simulink model "TestFun_2017"  (R2017a)
settings: Solver=VariableStepAuto  StartTime=0.0  StopTime=5  MaxStep=1e-3  RelTol=1e-3
undefined symbols (not defined in the file or in its folder): Evaluate_Trajectory
settings Model: Creator=Roberto Strada  LastModifiedBy=Davide
settings DataIOCC: ReturnWorkspaceOutputs=on
settings SFSimCC: SimUseLocalCustomCode=on
settings RTWCC: RTWUseLocalCustomCode=on

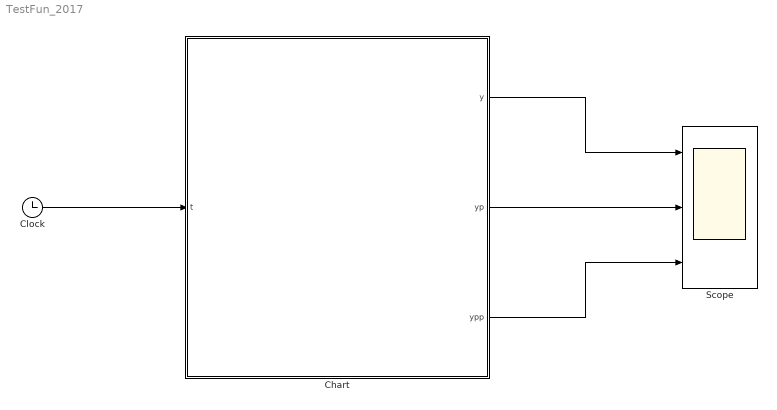
== system TestFun_2017 ==
  Chart : Stateflow chart  TreatAsAtomicUnit=on
  Clock : Clock
  Scope : Scope  NumInputPorts=3
  wires:
  Clock/1 -> Chart/1(t)
  Chart/2(yp) -> Scope/2
  Chart/1(y) -> Scope/1
  Chart/3(ypp) -> Scope/3

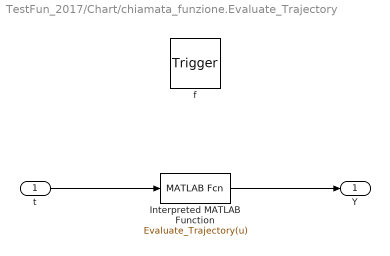
== system TestFun_2017/Chart/chiamata_funzione.Evaluate_Trajectory ==
  t : Inport  OutDataTypeStr=double  PortDimensions=1
  f : TriggerPort  TriggerType=function-call  VariantControl=(inherit)
      settings: CopyFcn=Stateflow.SLINSF.SimulinkMan.removeBlockPreDeleteFcn  PreDeleteFcn=Stateflow.SLINSF.SimulinkMan.unsafePredeleteFcn
  Interpreted MATLAB Function : MATLABFcn  MATLABFcn=Evaluate_Trajectory(u)  OutputDimensions=3
  Y : Outport
  wires:
  t/1 -> Interpreted MATLAB Function/1
  Interpreted MATLAB Function/1 -> Y/1

== stateflow chart TestFun_2017/Chart ==
  state chiamata_funzione
    du:
    Y=Evaluate_Trajectory(t);
    y=Y(1);
    yp=Y(2);
    ypp=Y(3);
    state Y=Evaluate_Trajectory(t) [function]
  (default) -> chiamata_funzione
  data: t function_input double size=1; Y function_output; t input; y output; yp output; ypp output; Y local
